simulink model "enabledTriggeredDiagram"  (R2015a)
settings: Solver=FixedStepDiscrete  SolverMode=SingleTasking  StartTime=0.0  StopTime=10.0  FixedStep=1  RelTol=1e-3
settings Model: CovMetricSettings=dwe  CovHtmlReporting=off  covSaveCumulativeToWorkspaceVar=off  CovSaveSingleToWorkspaceVar=off  CovExternalEMLEnable=on  Creator=hbourbou  LastModifiedBy=hbourbou
settings DataIOCC: LimitDataPoints=off  SaveFormat=Dataset
settings DebuggingCC: SFUnexpectedBacktrackingDiag=error  SFNoUnconditionalDefaultTransitionDiag=error
settings HardwareCC: ProdBitPerPointer=64  ProdLargestAtomicFloat=Float  ProdIntDivRoundTo=Zero  ProdEndianess=LittleEndian  ProdHWDeviceType=Specified
settings ModelReferenceCC: PropagateSignalLabelsOutOfModel=on
settings GRTTargetCC: TargetLangStandard=C99 (ISO)  GeneratePreprocessorConditionals=Use local settings

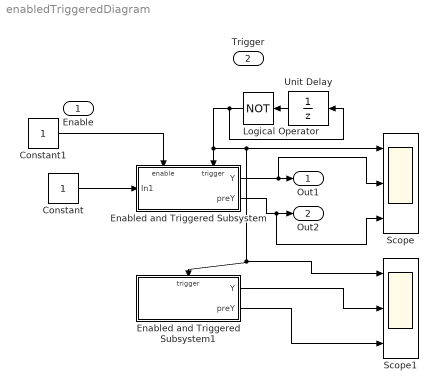
== system enabledTriggeredDiagram ==
  Enable : Inport  OutDataTypeStr=boolean
  Trigger : Inport  Port=2  OutDataTypeStr=boolean
  Constant : Constant
  Constant1 : Constant  OutDataTypeStr=boolean
  Enabled and Triggered Subsystem : Subsystem  TreatAsAtomicUnit=on
  Enabled and Triggered Subsystem1 : Subsystem  TreatAsAtomicUnit=on
  Logical Operator : Logic  Operator=NOT  AllPortsSameDT=off  OutDataTypeStr=boolean
  Scope : Scope  NumInputPorts=3
      settings: TimeRange=auto  MaxDataPoints=5000  SaveToWorkspace=off  SaveName=ScopeData  YMin=-0.125~-0.125~-0.125  YMax=1.125~11.125~11.125  SampleTime=-1
  Scope1 : Scope  NumInputPorts=3
      settings: TimeRange=auto  MaxDataPoints=5000  SaveToWorkspace=off  YMin=-0.125~-0.125~-0.125  YMax=1.125~11.125~11.125  SampleTime=-1
  Unit Delay : UnitDelay  InitialCondition=true  SampleTime=-1
  Out1 : Outport
  Out2 : Outport  Port=2
  wires:
  Constant/1 -> Enabled and Triggered Subsystem/1(In1)
  Enabled and Triggered Subsystem/1(Y) -> Scope/2, Out1/1
  Constant1/1 -> Enabled and Triggered Subsystem/Enable
  Logical Operator/1 -> Unit Delay/1, Enabled and Triggered Subsystem/Trigger, Scope1/1, Enabled and Triggered Subsystem1/Trigger, Scope/1
  Enabled and Triggered Subsystem/2(preY) -> Scope/3, Out2/1
  Unit Delay/1 -> Logical Operator/1
  Enabled and Triggered Subsystem1/1(Y) -> Scope1/2
  Enabled and Triggered Subsystem1/2(preY) -> Scope1/3

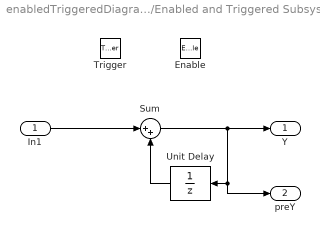
== system enabledTriggeredDiagram/Enabled and Triggered Subsystem ==
  In1 : Inport
  Enable : EnablePort  StatesWhenEnabling=reset
  Trigger : TriggerPort
  Sum : Sum  Inputs=|++
  Unit Delay : UnitDelay  SampleTime=-1
  Y : Outport  OutputWhenDisabled=reset  InitialOutput=10
  preY : Outport  Port=2  OutputWhenDisabled=reset  InitialOutput=10
  wires:
  In1/1 -> Sum/1
  Sum/1 -> preY/1, Unit Delay/1, Y/1
  Unit Delay/1 -> Sum/2

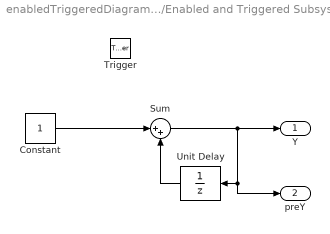
== system enabledTriggeredDiagram/Enabled and Triggered Subsystem1 ==
  Trigger : TriggerPort
  Constant : Constant
  Sum : Sum  Inputs=|++
  Unit Delay : UnitDelay  SampleTime=-1
  Y : Outport  OutputWhenDisabled=reset  InitialOutput=10
  preY : Outport  Port=2  OutputWhenDisabled=reset  InitialOutput=10
  wires:
  Constant/1 -> Sum/1
  Sum/1 -> preY/1, Unit Delay/1, Y/1
  Unit Delay/1 -> Sum/2
